simulink model "etc_plant_simple"  (R2024a)
settings: Solver=VariableStepAuto  StartTime=0.0  StopTime=20  RelTol=1e-3  EnableMultiTasking=on
PreLoadFcn:
  | % Throttle system parameters
  | etc_plant_data;
values from neighbouring files (symbols this model uses):
  J = 0.000245    [allParamValues.mat]
  Kd = 0.03    [allParamValues.mat]
  Km = 3    [allParamValues.mat]
  Ks = 0.2    [allParamValues.mat]
  theta_eq = 0.523598775598    [allParamValues.mat]
libraries: SignalEditorBlockLib x1
settings Model: LastModifiedBy=bneiswan
settings SolverCC: ZeroCrossControl=EnableAll  AlgebraicLoopSolver=TrustRegion  AutoInsertRateTranBlk=on
settings DataIOCC: SaveState=on
settings OptimizationCC: ReuseModelBlockBuffer=off  ExpressionDepthLimit=2147483647  InitFltsAndDblsToZero=on  LifeSpan=1  EfficientTunableParamExpr=on
settings DebuggingCC: UnconnectedInputMsg=warning  UnconnectedOutputMsg=warning  UnconnectedLineMsg=warning  PregeneratedLibrarySubsystemCodeDiagnostic=none  SubsystemReferenceDiagnosticForUnitTest=warning
settings HardwareCC: ProdBitPerPointer=32  ProdBitPerSizeT=32  ProdBitPerPtrDiffT=32  ProdLargestAtomicFloat=None  ProdIntDivRoundTo=Undefined  ProdEndianess=Unspecified  ProdWordSize=32  ProdHWDeviceType=32-bit Generic
settings ModelReferenceCC: EnableRefExpFcnMdlSchedulingChecks=on  PropagateSignalLabelsOutOfModel=off
settings SFSimCC: SimUseLocalCustomCode=off  MATLABDynamicMemAlloc=off
settings RTWCC: Description=RTW Embedded Coder (no auto configuration)  SystemTargetFile=ert.tlc  GenCodeOnly=on  TemplateMakefile=ert_default_tmf  RTWUseLocalCustomCode=off  GPUComputeCapability=3.5  DLArmComputeVersion=19.05
settings CodeAppCC: IgnoreCustomStorageClasses=off  CustomSymbolStrType=$N$R$M  StateflowObjectComments=on  InternalIdentifier=Classic
settings ERTTargetCC: TargetFcnLib=ansi_tfl_tmw.mat  MultiwordLength=2048  GenerateSampleERTMain=on  ERTCustomFileTemplate=example_file_process.tlc  ConvertIfToSwitch=off  SuppressUnreachableDefaultCases=off
settings ConfigComp: CovMetricSettings=dw  CovSaveCumulativeToWorkspaceVar=on  CovSaveSingleToWorkspaceVar=on  CovExternalEMLEnable=off  CovSFcnEnable=off

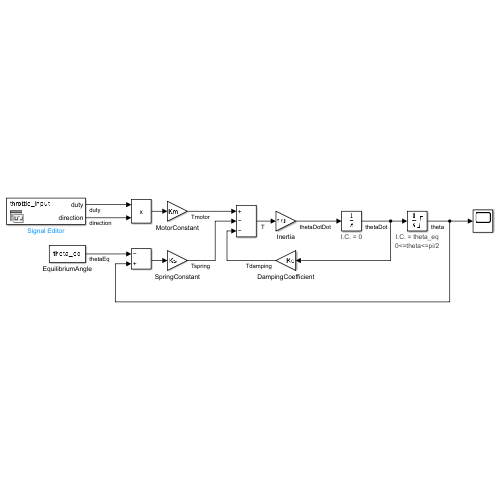
[thumbnail: Simulink's stored preview of the top-level diagram]
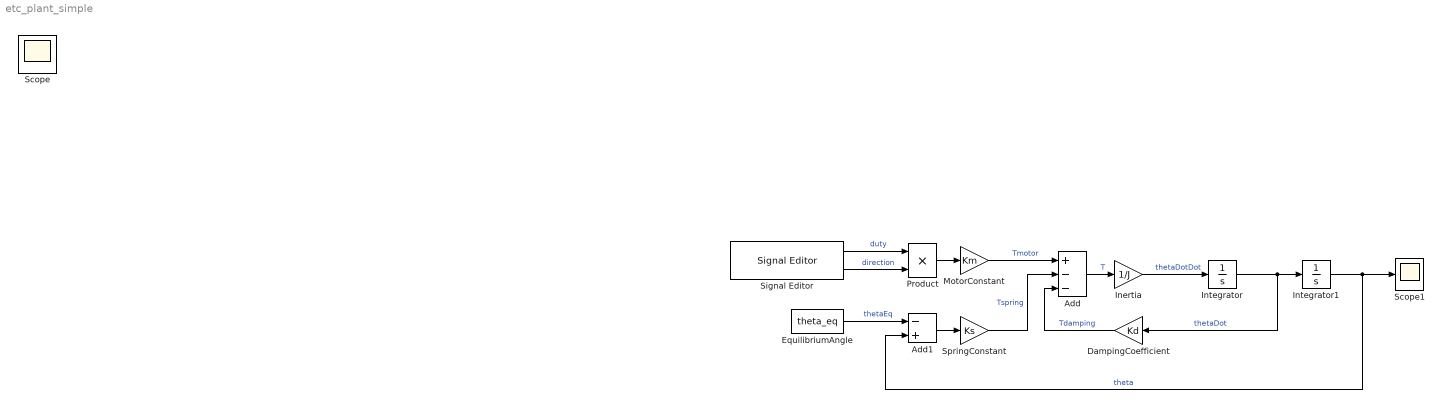
== system etc_plant_simple ==
  Add : Sum  Inputs=+--
  Add1 : Sum  Inputs=-+
  DampingCoefficient : Gain  Gain=Kd
  EquilibriumAngle : Constant  Value=theta_eq
  Inertia : Gain  Gain=1/J
  Integrator : Integrator
      settings: AttributesFormatString=I.C. = %<InitialCondition>
  Integrator1 : Integrator  InitialCondition=theta_eq  LimitOutput=on  UpperSaturationLimit=pi/2  LowerSaturationLimit=0
      settings: AttributesFormatString=|
      | I.C. = %<InitialCondition>
      | %<LowerSaturationLimit><=theta<=%<UpperSaturationLimit>
  MotorConstant : Gain  Gain=Km
  Product : Product
  Scope1 : Scope
  Signal Editor : SignalEditorBlockLib/Signal Editor  FileName=throttle_input_data.mat  ActiveScenario=throttle_input  ActiveSignal=duty  IsBus=off  OutputBusObjectStr=Bus: BusObject  SampleTime=0  Interpolate=off  ZeroCross=off  OutputAfterFinalValue=Setting to zero  Unit=inherit  PreserveSignalName=on  ApplySigPropsToAllScenarios=on  ApplySigPropsToAllSignals=off
  SpringConstant : Gain  Gain=Ks
  Scope : Scope
  wires:
  DampingCoefficient/1 -> Add/3  "Tdamping"
  Integrator/1 -> Integrator1/1, DampingCoefficient/1  "thetaDot"
  Add/1 -> Inertia/1  "T"
  Inertia/1 -> Integrator/1  "thetaDotDot"
  MotorConstant/1 -> Add/1  "Tmotor"
  SpringConstant/1 -> Add/2  "Tspring"
  Add1/1 -> SpringConstant/1
  Signal Editor/1 -> Product/1  "duty"
  Signal Editor/2 -> Product/2  "direction"
  Product/1 -> MotorConstant/1
  EquilibriumAngle/1 -> Add1/1  "thetaEq"
  Integrator1/1 -> Add1/2, Scope1/1  "theta"
